simulink model "Torque_PIL"  (R2023b)
settings: Solver=FixedStepAuto  StartTime=0.0  StopTime=300  RelTol=1e-3  EnableMultiTasking=on
values from neighbouring files (symbols this model uses):
  alpha = exp(-Tfs/Ts)    [model_approximation.m]
  k = 0.85    [torque.m]
  Ts = 0.005    [attempt.m]    (also in model_approximation.m; tuning.m)
libraries: mbedblockslib x4, cstblocks x1, stm_qeplib x1
settings Model: ExtModeTrigDuration=10  Creator=giova  LastModifiedBy=david
settings OptimizationCC: EnhancedBackFolding=on  PassReuseOutputArgsAs=Individual arguments  ZeroExternalMemoryAtStartup=off  ZeroInternalMemoryAtStartup=off  MaxStackSize=64  OptimizeBlockOrder=speed  DifferentSizesBufferReuse=on  OptimizationCustomize=off  EfficientTunableParamExpr=on
settings DebuggingCC: ParameterTunabilityLossMsg=error
settings HardwareCC: ProdBitPerPointer=32  ProdBitPerSizeT=32  ProdBitPerPtrDiffT=32  ProdLargestAtomicInteger=Long  ProdLargestAtomicFloat=Double  ProdWordSize=32  ProdLongLongMode=on  ProdHWDeviceType=ARM Compatible->ARM Cortex
settings SFSimCC: MATLABDynamicMemAlloc=off
settings RTWCC: Description=Embedded Coder  SystemTargetFile=ert.tlc  HardwareBoard=STM32 Nucleo F401RE  TemplateMakefile=ert_default_tmf  Toolchain=GNU Tools for ARM Embedded Processors
settings CodeAppCC: ForceParamTrailComments=on  IgnoreCustomStorageClasses=off  OperatorAnnotations=on  SimulinkDataObjDesc=on  SFDataObjDesc=on  InsertBlockDesc=on
settings ERTTargetCC: ExtModeTransport=3  ExtModeStaticAlloc=on  ExtModeStaticAllocSize=2000  ExtModeMexFile=ext_xcp  ExtModeIntrfLevel=Level2 - Open

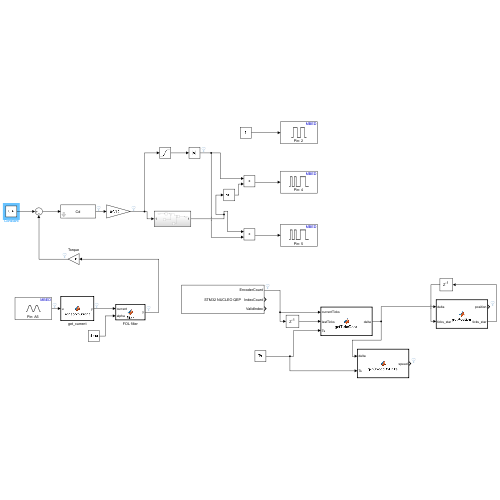
[thumbnail: Simulink's stored preview of the top-level diagram]
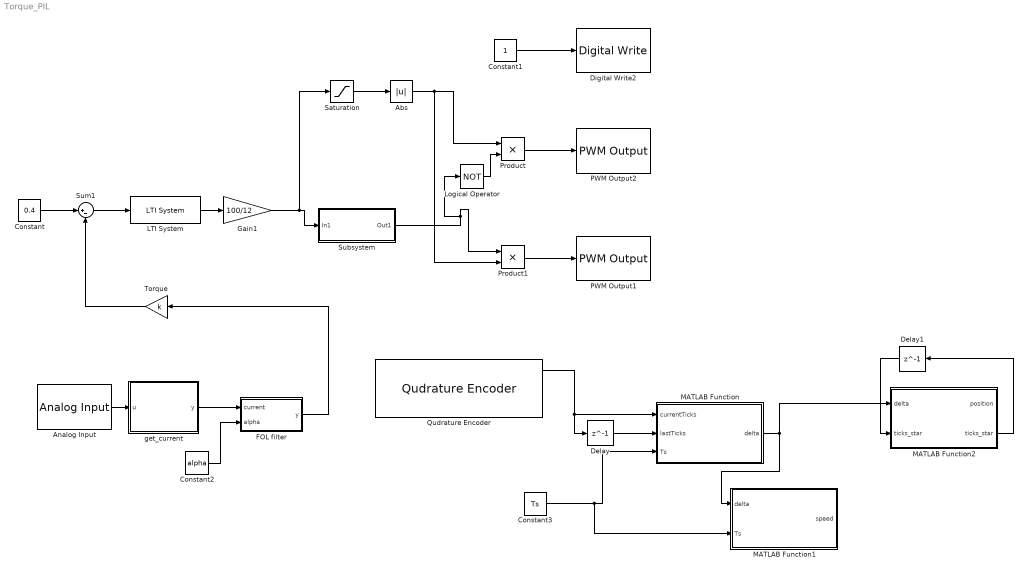
== system Torque_PIL ==
  Abs : Abs  SaturateOnIntegerOverflow=off
  Analog Input : mbedblockslib/Analog Input  Pin=A5  ReadResultsOnly=off  ConversionTriggerSource=Software  ExternalTriggerType=uint32( 0 )  OutputDataType=double  EnableConversionCompleteNotify=off  EnableOuputStatus=off  SampleTime=Ts
      settings: LibrarySourceBlock=stmnucleorootlib/Common/Analog Input
  Constant : Constant  Value=0.4
  Constant1 : Constant
  Constant2 : Constant  Value=alpha
  Constant3 : Constant  Value=Ts
  Delay : Delay  DelayLength=1  SampleTime=Ts
  Delay1 : Delay  DelayLength=1  SampleTime=Ts
  Digital Write2 : mbedblockslib/Digital Write  Pin=2  Direction=output
      settings: LibrarySourceBlock=stmnucleorootlib/Common/Digital Write
  FOL filter : MATLAB Function  TreatAsAtomicUnit=on
  Gain1 : Gain  Gain=100/12
  LTI System : cstblocks/LTI System  sys=Cd  IC=[]  PadeOrder=0
  Logical Operator : Logic  Operator=NOT  AllPortsSameDT=off  OutDataTypeStr=boolean
  MATLAB Function : MATLAB Function  TreatAsAtomicUnit=on
  MATLAB Function1 : MATLAB Function  TreatAsAtomicUnit=on
  MATLAB Function2 : MATLAB Function  TreatAsAtomicUnit=on
  PWM Output1 : mbedblockslib/PWM Output  Pin=5  EnableInputFrequency=off  InitialFrequency=2000  InitialDutyCycle=50  NotificationType=None
      settings: LibrarySourceBlock=stmnucleorootlib/Common/PWM Output
  PWM Output2 : mbedblockslib/PWM Output  Pin=4  EnableInputFrequency=off  InitialFrequency=2000  InitialDutyCycle=50  NotificationType=None
      settings: LibrarySourceBlock=stmnucleorootlib/Common/PWM Output
  Product : Product
  Product1 : Product
  Qudrature Encoder : stm_qeplib/Qudrature Encoder  SampleTime=Ts
  Saturation : Saturate  UpperLimit=100  LowerLimit=-100
  Subsystem : Subsystem
  Sum1 : Sum  Inputs=|+-
  Torque : Gain  Gain=k
  get_current : MATLAB Function  TreatAsAtomicUnit=on
  wires:
  Constant/1 -> Sum1/1
  Sum1/1 -> LTI System/1
  Torque/1 -> Sum1/2
  Saturation/1 -> Abs/1
  Logical Operator/1 -> Product/2
  Constant1/1 -> Digital Write2/1
  Abs/1 -> Product1/2, Product/1
  Product1/1 -> PWM Output1/1
  Product/1 -> PWM Output2/1
  Gain1/1 -> Saturation/1, Subsystem/1(In1)
  Subsystem/1(Out1) -> Logical Operator/1, Product1/1
  LTI System/1 -> Gain1/1
  Analog Input/1 -> get_current/1(u)
  get_current/1(y) -> FOL filter/1(current)
  Constant2/1 -> FOL filter/2(alpha)
  FOL filter/1(y) -> Torque/1
  MATLAB Function2/2(ticks_star) -> Delay1/1
  Qudrature Encoder/1 -> MATLAB Function/1(currentTicks), Delay/1
  Constant3/1 -> MATLAB Function1/2(Ts), MATLAB Function/3(Ts)
  Delay/1 -> MATLAB Function/2(lastTicks)
  MATLAB Function/1(delta) -> MATLAB Function1/1(delta), MATLAB Function2/1(delta)
  Delay1/1 -> MATLAB Function2/2("ticks_star ")

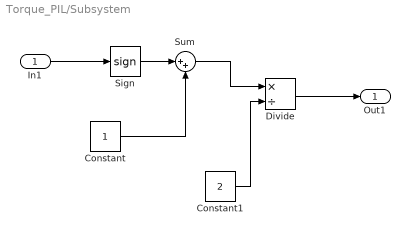
== system Torque_PIL/Subsystem ==
  In1 : Inport
  Constant : Constant
  Constant1 : Constant  Value=2
  Divide : Product  Inputs=*/
  Sign : Signum
  Sum : Sum  Inputs=|++
  Out1 : Outport
  wires:
  Constant/1 -> Sum/2
  In1/1 -> Sign/1
  Sign/1 -> Sum/1
  Sum/1 -> Divide/1
  Constant1/1 -> Divide/2
  Divide/1 -> Out1/1

== matlab function Torque_PIL/MATLAB Function1 ==
  data: delta input; speed output; Ts input
function speed = getSpeedByDelta(delta, Ts)
    speed = delta*60/(8400*Ts)

end

== matlab function Torque_PIL/MATLAB Function ==
  data: currentTicks input; delta output; lastTicks input; Ts input
function delta = getTicksDelta(currentTicks, lastTicks, Ts)

currentTicks = double(currentTicks);
lastTicks = double(lastTicks);

if abs(currentTicks-lastTicks) <= ceil(12600*Ts)
    delta = currentTicks-lastTicks
else
    if lastTicks > currentTicks
        delta = currentTicks+2^16-1-lastTicks;
    else
        delta = currentTicks-2^16+1-lastTicks;
    end
end

end

== matlab function Torque_PIL/MATLAB Function2 ==
  data: delta input; position output; ticks_star input; ticks_star output
function [position,ticks_star] = getPosition(delta, ticks_star)
    
    ticks_star = double(ticks_star+delta);

    completeTheta = 2*pi*ticks_star/(8400);

    position = sign(completeTheta)*mod(abs(completeTheta),2*pi);

end

== matlab function Torque_PIL/FOL filter ==
  data: current input; y output; alpha input
function y = filter(current, alpha)
    persistent current_old current_filtered_old;

    if isempty(current_old)
        current_old = current;
        current_filtered_old = 0;
    else
        current_temp = current;
        current = alpha*current_filtered_old + (1 - alpha) *current_old;
        current_old = current_temp;
        current_filtered_old = current;
    end

y = current;

== matlab function Torque_PIL/get_current ==
  data: u input; y output
function y = sensor2current(u)
    v_input = u*3.3;
    current = (1/0.185)*(v_input-2.5673);
y = current
